simulink model "Separately_Excited_DC_Motor"  (R2020a)
settings: Solver=VariableStepAuto  StartTime=0.0  StopTime=10.0  RelTol=1e-3
settings Model: Creator=Administrator  LastModifiedBy=Administrator

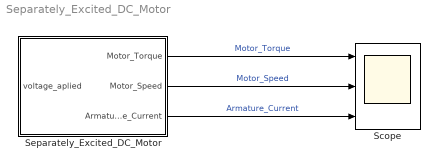
== system Separately_Excited_DC_Motor ==
  Scope : Scope  NumInputPorts=3
  Separately_Excited_DC_Motor : Subsystem  mask{La=.1, Ra=.5, Kphi=1.6, TL=20, B=.01, J=5}
      mask prompts: La "indectance (H)"; Ra "resactance(Ohm)"; TL "Torque Load(N.m)"; J "Moment of inertia(Kg.m)"
      mask DialogControl DescGroupVar Prompt: Separately Excited DC Motor
      mask DialogControl mohamend Prompt: This type of motors is used in trains and for automatic traction purposes.
  wires:
  Separately_Excited_DC_Motor/3(Armature_Current) -> Scope/3  "Armature_Current"
  Separately_Excited_DC_Motor/1(Motor_Torque) -> Scope/1  "Motor_Torque"
  Separately_Excited_DC_Motor/2(Motor_Speed) -> Scope/2  "Motor_Speed"

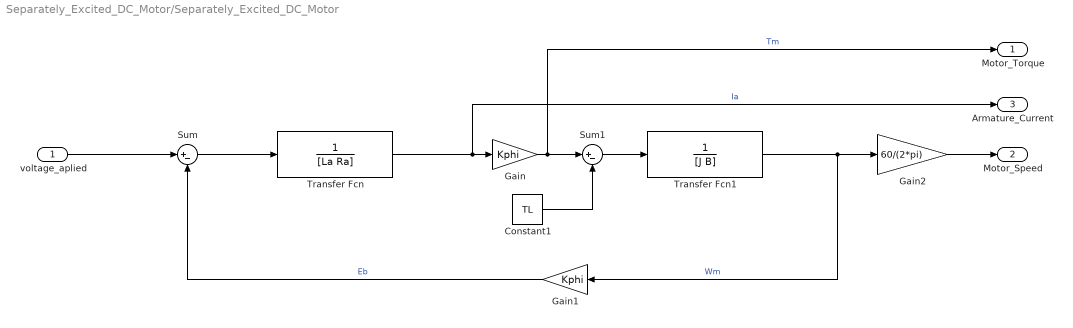
== system Separately_Excited_DC_Motor/Separately_Excited_DC_Motor ==
  voltage_aplied : Inport
  Constant1 : Constant  Value=TL
  Gain : Gain  Gain=Kphi
  Gain1 : Gain  Gain=Kphi
  Gain2 : Gain  Gain=60/(2*pi)
  Sum : Sum  Inputs=|+-
  Sum1 : Sum  Inputs=|+-
  Transfer Fcn : TransferFcn  Denominator=[La Ra]
  Transfer Fcn1 : TransferFcn  Denominator=[J B]
  Motor_Torque : Outport
  Motor_Speed : Outport  Port=2
  Armature_Current : Outport  Port=3
  wires:
  Gain2/1 -> Motor_Speed/1
  Transfer Fcn1/1 -> Gain2/1, Gain1/1  "Wm"
  Sum1/1 -> Transfer Fcn1/1
  Constant1/1 -> Sum1/2
  Gain/1 -> Sum1/1, Motor_Torque/1  "Tm"
  Transfer Fcn/1 -> Armature_Current/1, Gain/1  "Ia"
  Sum/1 -> Transfer Fcn/1
  Gain1/1 -> Sum/2  "Eb"
  voltage_aplied/1 -> Sum/1
